simulink library "LiftMotionControlLibrary"  (R2021b)
settings: Solver=VariableStepAuto  StartTime=0.0  StopTime=10.0  RelTol=1e-3
values from neighbouring files (symbols this model uses):
  floor_height = 3    [test_motion_law.m]
  gearbox = 1    [test_motion_law.m]
  max_load = 800    [test_motion_law.m]
  MaxAcc = 1    [test_motion_law.m]
  MaxJerk = 1    [test_motion_law.m]
  MaxVel = 2    [test_motion_law.m]
  MinVel = 0.2    [test_motion_law.m]
  motion_profile = 1    [test_motion_law.m]
  num_floors = 20    [test_motion_law.m]
  proximity_distance = 1    [test_motion_law.m]
  Ts = 1e-3    (= 0.001)    [test_motion_law.m]
undefined symbols (not defined in the file or in its folder): cabin_offset, Rp, sensor_height, waiting_time_close_brake, waiting_time_close_door, waiting_time_open_brake, waiting_time_open_door, waiting_time_steady_state
libraries: $bdroot x2, cstblocks x1
settings Model: Creator=manue  LastModifiedBy=manue

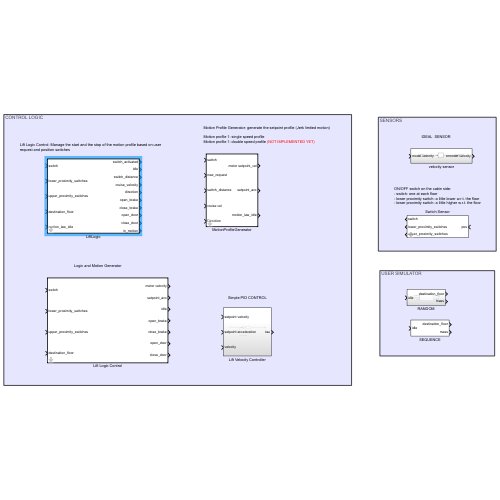
[thumbnail: Simulink's stored preview of the top-level diagram]
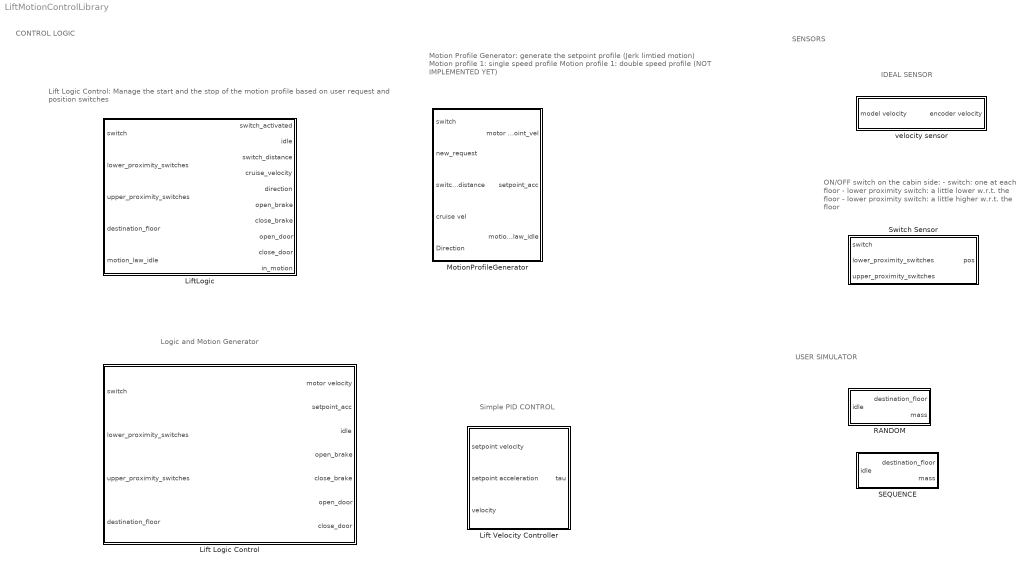
== system LiftMotionControlLibrary ==
  note: Logic and Motion Generator
  note: IDEAL SENSOR
  note: ON/OFF switch on the cabin side:
      | - switch: one at each floor
      | - lower proximity switch: a little lower w.r.t. the floor
      | - lower proximity switch: a little higher w.r.t. the floor
  note: SENSORS
  note: CONTROL LOGIC
  note: Simple PID CONTROL
  note: Motion Profile Generator: generate the setpoint profile (Jerk limtied motion)
      |
      | Motion profile 1: single speed profile
      | Motion profile 1: double speed profile (NOT IMPLEMENTED YET)
  note: Lift Logic Control: Manage the start and the stop of the motion profile based on user request and position switches
  note: USER SIMULATOR
  Lift Logic Control : Subsystem  TreatAsAtomicUnit=on  SystemSampleTime=Ts  mask{floor_height=floor_height, num_floors=num_floors, sensor_height=sensor_height, proximity_distance=proximity_distance, MinVel=MinVel, MaxVel=MaxVel, Ts=Ts, MaxAcc=MaxAcc, MaxJerk=MaxJerk, gearbox=gearbox, cabin_offset=cabin_offset, Rp=Rp, motion_profile=Profile 1: single speed, waiting_time_open_door=waiting_time_open_door, waiting_time_close_door=waiting_time_close_door, waiting_time_open_brake=waiting_time_open_brake, waiting_time_close_brake_copy=waiting_time_close_brake, waiting_time_steady_state=waiting_time_steady_state}
      mask prompts: floor_height "Floor Height"; num_floors "Number of floors"; sensor_height "Sensor Height"; proximity_distance "Distance of the proximity switches"; MinVel "Lower lift velocity"; MaxVel "Maximum lift velocity"; Ts "Sample period"; MaxAcc "Maximum acceleration"; MaxJerk "Maximum Jerk"; gearbox "gearbox ratio"; cabin_offset "Cabin offset compensation"; Rp "Pulley Radius"; motion_profile "Type of Motion Profile"; waiting_time_open_door "Time to open doors"; waiting_time_close_door "Time to close doors"; waiting_time_open_brake "Time to open brake"; waiting_time_close_brake_copy "Time to close brake"; waiting_time_steady_state "Time to reach zero velocity"
      mask TypeOptions motion_profile: Profile 1: single speed | Profile 2: multiple speed (not implmeneted yet)
  Lift Velocity Controller : Subsystem
  LiftLogic : Subsystem  TreatAsAtomicUnit=on  SystemSampleTime=Ts  mask{floor_height=floor_height, num_floors=num_floors, sensor_height=sensor_height, proximity_distance=proximity_distance, motion_profile=motion_profile, MinVel=MinVel, MaxVel=MaxVel, cabin_offset=cabin_offset, Ts=Ts, waiting_time_open_door=waiting_time_open_door, waiting_time_close_door=waiting_time_close_door, waiting_time_open_brake=waiting_time_open_brake, waiting_time_close_brake=waiting_time_close_brake, waiting_time_steady_state=waiting_time_steady_state}
      mask prompts: floor_height "Floor Height"; num_floors "Number of floors"; sensor_height "Sensor Height"; proximity_distance "Distance of the proximity switches"; motion_profile "Type of Motion Profile"; MinVel "Lower lift velocity"; MaxVel "Maximum lift velocity"; cabin_offset "Cabin offset compensation"; Ts "Sample period"; waiting_time_open_door "Time to open the doors"; waiting_time_close_door "Time to close the doors"; waiting_time_open_brake "Time to open the brake"; waiting_time_close_brake "Time to close the brake"; waiting_time_steady_state "Time to reach zero velocity"
  MotionProfileGenerator : Subsystem  TreatAsAtomicUnit=on  SystemSampleTime=Ts  mask{MaxAcc=MaxAcc, MaxJerk=MaxJerk, Ts=Ts, gearbox=gearbox, Rp=Rp, motion_profile=motion_profile}
      mask prompts: MaxAcc "Maximum acceleration"; MaxJerk "MaximumJerk"; Ts "Sample period"; gearbox "gearbox ratio"; Rp "Pulley Radius"; motion_profile "Type of Motion profile"
  RANDOM : Subsystem
  SEQUENCE : Subsystem  mask{sequence=[5 10 15 10]}
      mask prompts: sequence "Floor sequence"
  Switch Sensor : Subsystem  mask{floor_height=floor_height, num_floors=num_floors, proximity_distance=proximity_distance, sensor_height=sensor_height}
      mask prompts: floor_height "Floor Height"; num_floors "Number of floors"; proximity_distance "Distance of the proximity switches"; sensor_height "Sensor Height"
      mask help: switches return -1 if not activated, the number of floor if activated
  velocity sensor : Subsystem

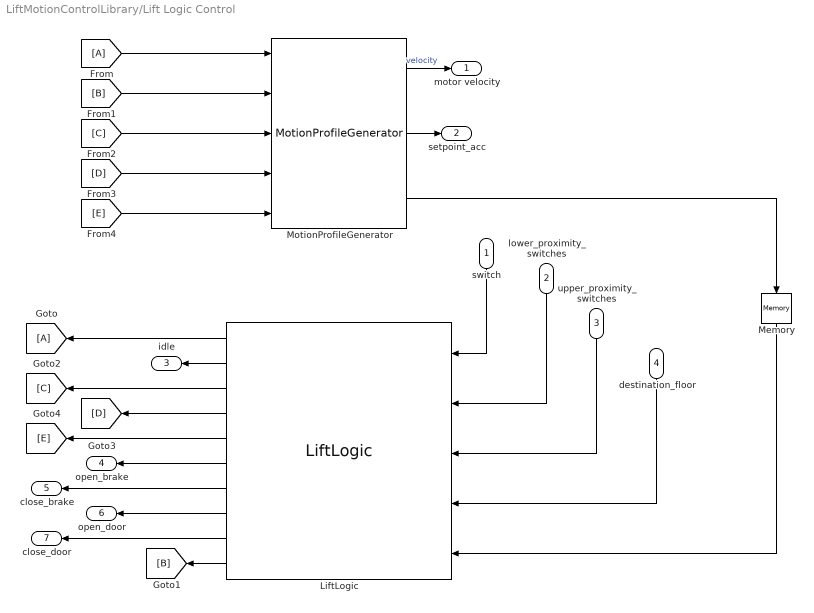
== system LiftMotionControlLibrary/Lift Logic Control ==
  switch : Inport
  lower_proximity_switches : Inport  Port=2
  upper_proximity_switches : Inport  Port=3
  destination_floor : Inport  Port=4
  LiftLogic : $bdroot/LiftLogic  floor_height=floor_height  num_floors=num_floors  sensor_height=sensor_height  proximity_distance=proximity_distance  motion_profile=motion_profile  MinVel=MinVel  MaxVel=MaxVel  cabin_offset=cabin_offset  Ts=Ts  waiting_time_open_door=waiting_time_open_door  waiting_time_close_door=waiting_time_close_door  waiting_time_open_brake=waiting_time_open_brake  waiting_time_close_brake=waiting_time_close_brake  waiting_time_steady_state=waiting_time_steady_state
  Memory : Memory  InheritSampleTime=on
  MotionProfileGenerator : $bdroot/MotionProfileGenerator  MaxAcc=MaxAcc  MaxJerk=MaxJerk  Ts=Ts  gearbox=gearbox  Rp=Rp  motion_profile=motion_profile
  motor velocity : Outport
  setpoint_acc : Outport  Port=2
  idle : Outport  Port=3
  open_brake : Outport  Port=4
  close_brake : Outport  Port=5
  open_door : Outport  Port=6
  close_door : Outport  Port=7
  wires:
  [E] -> MotionProfileGenerator/5
  LiftLogic/5 -> [E]
  [D] -> MotionProfileGenerator/4
  LiftLogic/4 -> [D]
  [C] -> MotionProfileGenerator/3
  LiftLogic/3 -> [C]
  LiftLogic/2 -> idle/1
  [A] -> MotionProfileGenerator/1
  LiftLogic/1 -> [A]
  Memory/1 -> LiftLogic/5
  MotionProfileGenerator/3 -> Memory/1
  destination_floor/1 -> LiftLogic/4
  lower_proximity_switches/1 -> LiftLogic/2
  switch/1 -> LiftLogic/1
  MotionProfileGenerator/1 -> motor velocity/1  "velocity"
  MotionProfileGenerator/2 -> setpoint_acc/1
  upper_proximity_switches/1 -> LiftLogic/3
  [B] -> MotionProfileGenerator/2
  LiftLogic/10 -> [B]
  LiftLogic/9 -> close_door/1
  LiftLogic/8 -> open_door/1
  LiftLogic/7 -> close_brake/1
  LiftLogic/6 -> open_brake/1

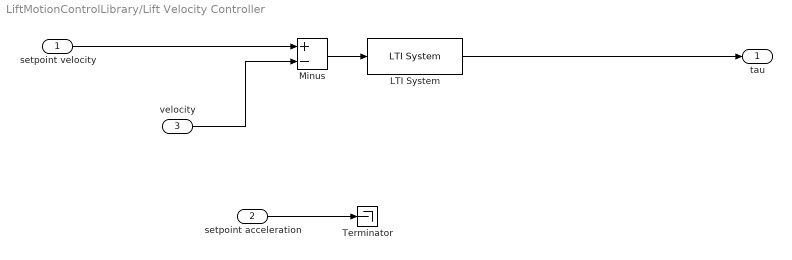
== system LiftMotionControlLibrary/Lift Velocity Controller ==
  setpoint velocity : Inport
  setpoint acceleration : Inport  Port=2
  velocity : Inport  Port=3
  LTI System : cstblocks/LTI System  sys=ctrl  IC=[]
  Minus : Sum  Inputs=+-
  Terminator : Terminator
  tau : Outport
  wires:
  setpoint acceleration/1 -> Terminator/1
  velocity/1 -> Minus/2
  Minus/1 -> LTI System/1
  setpoint velocity/1 -> Minus/1
  LTI System/1 -> tau/1

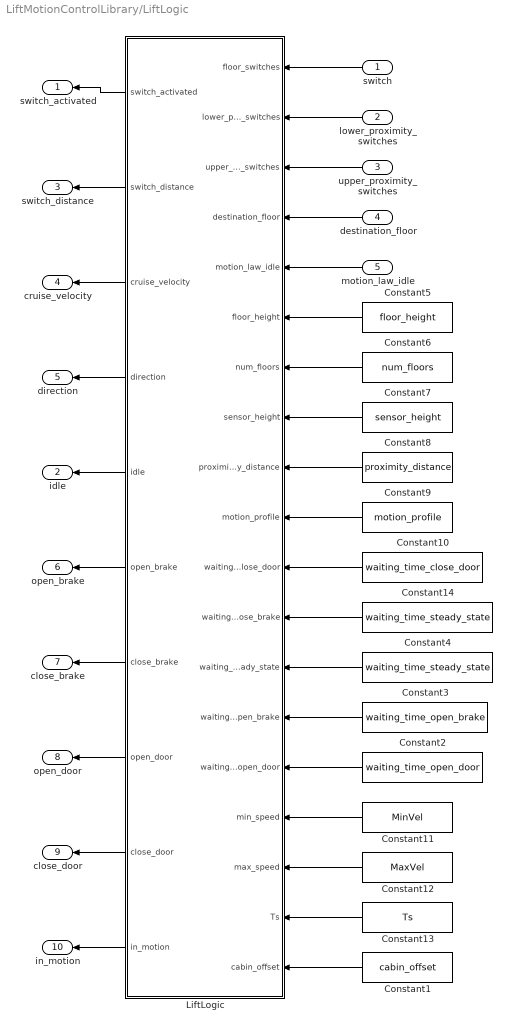
== system LiftMotionControlLibrary/LiftLogic ==
  switch : Inport
  lower_proximity_switches : Inport  Port=2
  upper_proximity_switches : Inport  Port=3
  destination_floor : Inport  Port=4
  motion_law_idle : Inport  Port=5
  Constant1 : Constant  Value=cabin_offset
  Constant10 : Constant  Value=waiting_time_close_door
  Constant11 : Constant  Value=MinVel
  Constant12 : Constant  Value=MaxVel
  Constant13 : Constant  Value=Ts
  Constant14 : Constant  Value=waiting_time_steady_state  VectorParams1D=off
  Constant2 : Constant  Value=waiting_time_open_door
  Constant3 : Constant  Value=waiting_time_open_brake
  Constant4 : Constant  Value=waiting_time_steady_state  VectorParams1D=off
  Constant5 : Constant  Value=floor_height
  Constant6 : Constant  Value=num_floors
  Constant7 : Constant  Value=sensor_height
  Constant8 : Constant  Value=proximity_distance
  Constant9 : Constant  Value=motion_profile
  LiftLogic : MATLAB Function  TreatAsAtomicUnit=on
  switch_activated : Outport  OutDataTypeStr=boolean
  idle : Outport  Port=2
  switch_distance : Outport  Port=3
  cruise_velocity : Outport  Port=4
  direction : Outport  Port=5
  open_brake : Outport  Port=6
  close_brake : Outport  Port=7
  open_door : Outport  Port=8
  close_door : Outport  Port=9
  in_motion : Outport  Port=10
  wires:
  LiftLogic/1(switch_activated) -> switch_activated/1
  Constant5/1 -> LiftLogic/6(floor_height)
  Constant11/1 -> LiftLogic/16(min_speed)
  Constant1/1 -> LiftLogic/19(cabin_offset)
  switch/1 -> LiftLogic/1(floor_switches)
  Constant12/1 -> LiftLogic/17(max_speed)
  Constant7/1 -> LiftLogic/8(sensor_height)
  Constant10/1 -> LiftLogic/11(waiting_time_close_door)
  LiftLogic/3(cruise_velocity) -> cruise_velocity/1
  upper_proximity_switches/1 -> LiftLogic/3(upper_proximity_switches)
  Constant13/1 -> LiftLogic/18(Ts)
  Constant8/1 -> LiftLogic/9(proximity_distance)
  motion_law_idle/1 -> LiftLogic/5(motion_law_idle)
  LiftLogic/4(direction) -> direction/1
  LiftLogic/5(idle) -> idle/1
  Constant6/1 -> LiftLogic/7(num_floors)
  LiftLogic/2(switch_distance) -> switch_distance/1
  destination_floor/1 -> LiftLogic/4(destination_floor)
  lower_proximity_switches/1 -> LiftLogic/2(lower_proximity_switches)
  Constant9/1 -> LiftLogic/10(motion_profile)
  Constant2/1 -> LiftLogic/15(waiting_time_open_door)
  Constant14/1 -> LiftLogic/12(waiting_time_close_brake)
  Constant4/1 -> LiftLogic/13(waiting_time_steady_state)
  Constant3/1 -> LiftLogic/14(waiting_time_open_brake)
  LiftLogic/6(open_brake) -> open_brake/1
  LiftLogic/7(close_brake) -> close_brake/1
  LiftLogic/8(open_door) -> open_door/1
  LiftLogic/9(close_door) -> close_door/1
  LiftLogic/10(in_motion) -> in_motion/1

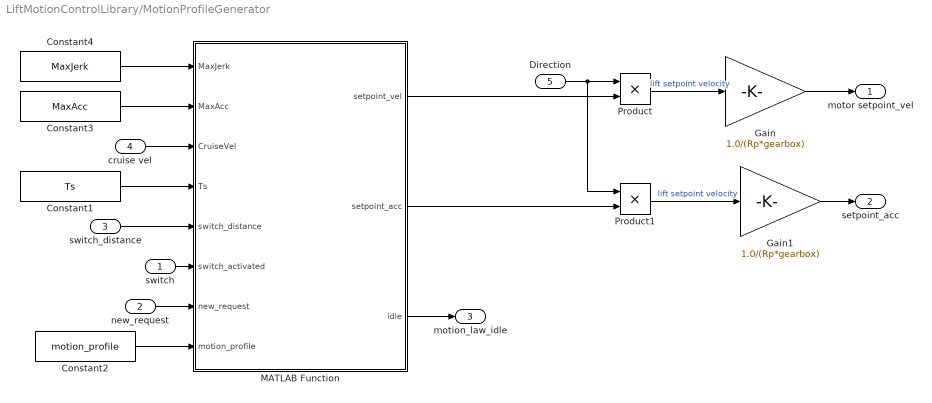
== system LiftMotionControlLibrary/MotionProfileGenerator ==
  switch : Inport
  new_request : Inport  Port=2
  switch_distance : Inport  Port=3
  cruise vel : Inport  Port=4
  Direction : Inport  Port=5
  Constant1 : Constant  Value=Ts
  Constant2 : Constant  Value=motion_profile
  Constant3 : Constant  Value=MaxAcc
  Constant4 : Constant  Value=MaxJerk
  Gain : Gain  Gain=1.0/(Rp*gearbox)
  Gain1 : Gain  Gain=1.0/(Rp*gearbox)
  MATLAB Function : MATLAB Function  TreatAsAtomicUnit=on
  Product : Product
  Product1 : Product
  motor setpoint_vel : Outport
  setpoint_acc : Outport  Port=2
  motion_law_idle : Outport  Port=3
  wires:
  new_request/1 -> MATLAB Function/7(new_request)
  MATLAB Function/3(idle) -> motion_law_idle/1
  Gain/1 -> motor setpoint_vel/1
  Product/1 -> Gain/1  "lift setpoint velocity"
  Direction/1 -> Product1/1, Product/1
  MATLAB Function/1(setpoint_vel) -> Product/2
  MATLAB Function/2(setpoint_acc) -> Product1/2
  Constant4/1 -> MATLAB Function/1(MaxJerk)
  Constant3/1 -> MATLAB Function/2(MaxAcc)
  switch/1 -> MATLAB Function/6(switch_activated)
  Constant1/1 -> MATLAB Function/4(Ts)
  switch_distance/1 -> MATLAB Function/5(switch_distance)
  cruise vel/1 -> MATLAB Function/3(CruiseVel)
  Gain1/1 -> setpoint_acc/1
  Product1/1 -> Gain1/1  "lift setpoint velocity"
  Constant2/1 -> MATLAB Function/8(motion_profile)

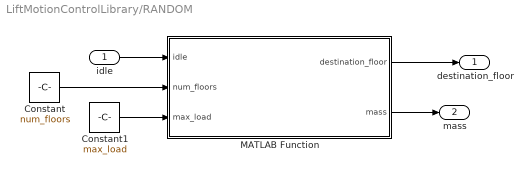
== system LiftMotionControlLibrary/RANDOM ==
  idle : Inport
  Constant : Constant  Value=num_floors
  Constant1 : Constant  Value=max_load
  MATLAB Function : MATLAB Function  TreatAsAtomicUnit=on
  destination_floor : Outport  OutDataTypeStr=double
  mass : Outport  Port=2  OutDataTypeStr=double
  wires:
  idle/1 -> MATLAB Function/1(idle)
  Constant/1 -> MATLAB Function/2(num_floors)
  Constant1/1 -> MATLAB Function/3(max_load)
  MATLAB Function/1(destination_floor) -> destination_floor/1
  MATLAB Function/2(mass) -> mass/1

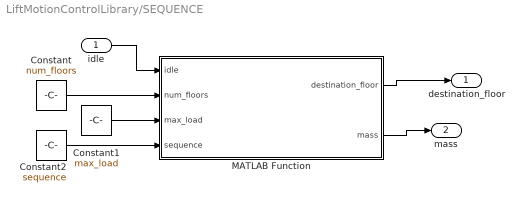
== system LiftMotionControlLibrary/SEQUENCE ==
  idle : Inport
  Constant : Constant  Value=num_floors
  Constant1 : Constant  Value=max_load
  Constant2 : Constant  Value=sequence
  MATLAB Function : MATLAB Function  TreatAsAtomicUnit=on
  destination_floor : Outport  OutDataTypeStr=double
  mass : Outport  Port=2  OutDataTypeStr=double
  wires:
  MATLAB Function/2(mass) -> mass/1
  MATLAB Function/1(destination_floor) -> destination_floor/1
  Constant1/1 -> MATLAB Function/3(max_load)
  Constant/1 -> MATLAB Function/2(num_floors)
  idle/1 -> MATLAB Function/1(idle)
  Constant2/1 -> MATLAB Function/4(sequence)

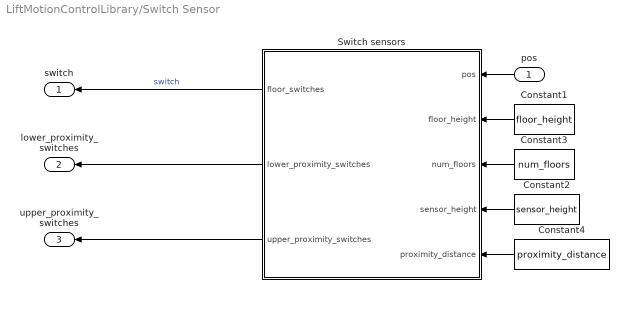
== system LiftMotionControlLibrary/Switch Sensor ==
  pos : Inport
  Constant1 : Constant  Value=floor_height
  Constant2 : Constant  Value=sensor_height
  Constant3 : Constant  Value=num_floors
  Constant4 : Constant  Value=proximity_distance
  Switch sensors : MATLAB Function  TreatAsAtomicUnit=on
  switch : Outport
  lower_proximity_switches : Outport  Port=2
  upper_proximity_switches : Outport  Port=3
  wires:
  Switch sensors/1(floor_switches) -> switch/1  "switch"
  pos/1 -> Switch sensors/1(pos)
  Constant1/1 -> Switch sensors/2(floor_height)
  Constant3/1 -> Switch sensors/3(num_floors)
  Constant4/1 -> Switch sensors/5(proximity_distance)
  Constant2/1 -> Switch sensors/4(sensor_height)
  Switch sensors/3(upper_proximity_switches) -> upper_proximity_switches/1
  Switch sensors/2(lower_proximity_switches) -> lower_proximity_switches/1

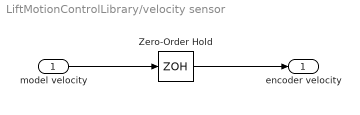
== system LiftMotionControlLibrary/velocity sensor ==
  model velocity : Inport
  Zero-Order Hold : ZeroOrderHold  SampleTime=Ts
  encoder velocity : Outport
  wires:
  model velocity/1 -> Zero-Order Hold/1
  Zero-Order Hold/1 -> encoder velocity/1

== matlab function LiftMotionControlLibrary/SEQUENCE/MATLAB Function ==
  data: idle input; destination_floor output; num_floors input; max_load input; mass output double; sequence input
function [destination_floor,mass]  = simulatePeople(idle,num_floors,max_load,sequence)

persistent destination_internal mass_internal idx_sequence
if isempty(destination_internal)
    destination_internal=0;
    mass_internal=0.0;
    idx_sequence=1;
end

if (idle)
    if (idx_sequence>length(sequence))
        idx_sequence=1;
    end
    destination_internal=sequence(idx_sequence);
    % mass variation for each cycles +/- 400 kg
    mass_internal=min(max(0,mass_internal+(2*rand-1)*80*5),max_load); 
    idx_sequence=idx_sequence+1;

end
destination_floor=destination_internal;
mass=mass_internal;

== matlab function LiftMotionControlLibrary/Switch Sensor/Switch sensors ==
  data: pos input; floor_switches output; floor_height input; num_floors input; sensor_height input; proximity_distance input; lower_proximity_switches output; upper_proximity_switches output
function [floor_switches,lower_proximity_switches,upper_proximity_switches]=SwitchPosition(pos,floor_height,num_floors,sensor_height,proximity_distance)
% switches return -1 if not activated, the number of floor if activated

floor_switches=-1;
lower_proximity_switches=-1;
upper_proximity_switches=-1;
for floor_index=0:num_floors

    % floor switch
    switch_pos=floor_index*floor_height;
    if (pos<=switch_pos && (pos+sensor_height)>=(switch_pos))
        floor_switches=floor_index;
    end

    % lower proximity switch
    switch_pos=floor_index*floor_height+sensor_height-proximity_distance;
    if (pos<=switch_pos && (pos+sensor_height)>=(switch_pos))
        lower_proximity_switches=floor_index;
    end
    
    % upper proximity switch
    switch_pos=floor_index*floor_height+proximity_distance;
    if (pos<=switch_pos && (pos+sensor_height)>=(switch_pos))
        upper_proximity_switches=floor_index;
    end
end

== matlab function LiftMotionControlLibrary/MotionProfileGenerator/MATLAB Function ==
  data: MaxJerk input; setpoint_vel output; MaxAcc input; CruiseVel input; Ts input; switch_distance input; switch_activated input; setpoint_acc output; new_request input; idle output boolean; motion_profile input
function [setpoint_vel,setpoint_acc,idle]=MotionLaw(MaxJerk,MaxAcc,CruiseVel,Ts,switch_distance,switch_activated,new_request,motion_profile)

persistent state vel acc pos
if isempty(state)
    state=0;
    vel=0;
    acc=0;
    pos=0;
end

% compute deceleration distance: 
% case 1: the maximum acceleration is reached
% case 2: the maximum acceleration is not reached
if (CruiseVel^(1/2)*MaxJerk^(1/2)>MaxAcc) % case 1
    deceleration_distance=(CruiseVel*(MaxAcc^2 + CruiseVel*MaxJerk))/(2*MaxAcc*MaxJerk);
else % case 2
    deceleration_distance =CruiseVel^(3/2)/MaxJerk^(1/2);
end

if (state==1)  %increase acceleration
    jerk=MaxJerk;
elseif (state==2) % max acceleration
    jerk=0;
elseif (state==3) % decrease acceleration
    jerk=-MaxJerk;
elseif (state==4) % keep cruise velocity
    jerk=0;
elseif (state==5) % kep cruise velocity, switch has been triggered
    jerk=0;
elseif (state==6) % decrease acceleration (to slow down speed)
    jerk=-MaxJerk;
elseif (state==7) % max negative acceleration (to slow down speed)
    jerk=0;
elseif (state==8) % increase acceleration (to return to null acceleration)
    jerk=MaxJerk;

elseif state==11 % decrease acceleration (to reach low speed)  PROFILE==2
    jerk=-MaxJerk;
elseif state==12 % max negative acceleration (to reach low speed)  PROFILE==2
    jerk=0;
elseif state==13 % increase acceleration (to return to null acceleration)  PROFILE==2
    jerk=MaxJerk;
elseif (state==14) % keep cruise velocity
    jerk=0;
else % steaty-state case
    jerk=0;
    vel=0;
    acc=0;

end


pos=pos+vel*Ts+0.5*acc*Ts^2+1.0/6.0*jerk*Ts^3; % traveled distance
vel=vel+acc*Ts+0.5*Ts*Ts*jerk; % velocity
acc=acc+Ts*jerk; % acceleration

limit_velocity=CruiseVel-acc^2/(2*MaxJerk); % velocity limit to start removing accelaration to reach cruise velocity
limit_velocity_profile2=CruiseVel+acc^2/(2*MaxJerk); % velocity limit to start removing accelaration to reach low velocity
limit_velocity_final=acc^2/(2*MaxJerk); % velocity limit to start removing accelaration to reach null velocity

%% state machine transition 
if (state==0 && new_request)
    state=1;
elseif (state==1 && acc>=MaxAcc) % max acceleration reached
    state=2;
    acc=min(acc,MaxAcc);
elseif ((state==2 || state==1) && vel>=limit_velocity) % limit velocity reached  (cruise velocity will be reached soon)
    state=3;
elseif (state==3 && acc<=0) % null acceleration reached
    state=4;
    acc=0;
elseif (state==4 && switch_activated) % switch has been triggered
    if (motion_profile==1)
        state=5;
    else
        state=11;
    end
    pos=0;
elseif (state==5 && pos>=(switch_distance-deceleration_distance)) % time to slow down
    state=6;
elseif (state==6 && acc<=-MaxAcc) % negative max acceleration reached
    state=7;
    acc=max(acc,-MaxAcc);
elseif ((state==7 || state==6) && vel<=limit_velocity_final) % limit acceleration to stop motion is reached
    state=8;
elseif (state==8 && vel<=0) % steady state reached
    state=0;
    vel=0;
    acc=0;


elseif (state==11 && acc<=-MaxAcc)
    state=12;
    acc=max(acc,-MaxAcc);
elseif ((state==11 || state==12)  && vel<=limit_velocity_profile2)
    state=13;
elseif (state==13 && vel<=CruiseVel) % steady state reached
    state=14;
    vel=CruiseVel;
    acc=0;
elseif (state==14 && switch_activated) % switch has been triggered
    state=5;
    pos=0;
end

idle=state==0;
setpoint_vel=vel;
setpoint_acc=acc;

== matlab function LiftMotionControlLibrary/LiftLogic/LiftLogic ==
  data: floor_switches input; switch_activated output; lower_proximity_switches input; upper_proximity_switches input; destination_floor input; motion_law_idle input; floor_height input; num_floors input; sensor_height input; proximity_distance input; motion_profile input; waiting_time_close_door input; waiting_time_close_brake input; waiting_time_steady_state input; waiting_time_open_brake input; waiting_time_open_door input; min_speed input; max_speed input; Ts input; switch_distance output; cruise_velocity output; direction output; idle output; cabin_offset input; open_brake output; close_brake output; open_door output; close_door output; in_motion output
function [switch_activated,switch_distance,cruise_velocity,direction,idle,open_brake,close_brake,open_door,close_door,in_motion]=LiftLogic(floor_switches,...
    lower_proximity_switches,...
    upper_proximity_switches,...
    destination_floor,...
    motion_law_idle,...
    floor_height,...
    num_floors,...
    sensor_height,...
    proximity_distance,...
    motion_profile,...
    waiting_time_close_door,...
    waiting_time_close_brake,...
    waiting_time_steady_state,...
    waiting_time_open_brake,...
    waiting_time_open_door,...
    min_speed,...
    max_speed,...
    Ts,...
    cabin_offset)

persistent req_floor state start_floor time cruise_velocity_internal direction_internal open_brake_cmd_internal open_door_internal close_brake_cmd_internal close_door_internal

if isempty(req_floor)
    if floor_switches>=0 % lift is parked in one floor at the beginning
        start_floor=floor_switches;
    else % abnormal behaviour lift in not parked in one floor at the beginning, go to the last floor
        start_floor=-1;
        destination_floor=num_floors;
    end
    req_floor=start_floor;
    state=0;
    time=0;
    cruise_velocity_internal=0;
    direction_internal=0;

    open_brake_cmd_internal=true;
    open_door_internal=false;
    close_brake_cmd_internal=false;
    close_door_internal=false;
end

switch_activated=false;
switch_distance=0;
idle=false;
% state:
% 0 IDLE
% 1 close the door
% 2 open the break
% 3 LIFT IS MOVING
% 4 LIFT IS MOVING AT LOW VELOCITY
% 5 STOPPING
% 6 close the break
% 7 open the door

% ACTIONS

if state==3
    if (direction_internal>0)
        switch_activated=floor_switches==(req_floor-1); % the top of the cabin reaches the floor switch
        switch_distance=floor_height+sensor_height+cabin_offset;
    else
        switch_activated=floor_switches==(req_floor+1); % the bottom of the cabin reaches the upper floor switch
        switch_distance=floor_height+cabin_offset;
    end
elseif state==4
    if (direction_internal>0)
        switch_activated=lower_proximity_switches==(req_floor); % the top of the cabin reaches the floor switch
        switch_distance= proximity_distance + cabin_offset;
    else
        switch_activated=upper_proximity_switches==(req_floor); % the bottom of the cabin reaches the upper floor switch
        switch_distance=proximity_distance+cabin_offset;
    end
elseif state~=0
    time=time+Ts;
end


in_motion=false;

% TRANSITIONS
if (state==0 && (destination_floor~=start_floor))
    if ( (destination_floor>num_floors) || (destination_floor<0) )
        % you should not go here!
    else
        time=0;
        state=1;
        req_floor=destination_floor;
        close_door_internal=true;
            if abs(req_floor-start_floor)==1
                cruise_velocity_internal=min_speed;
            else
                cruise_velocity_internal=max_speed;
            end
            if (req_floor>start_floor)
                direction_internal=1;
            else
                direction_internal=-1;
            end

    end
elseif (state==1 && time>waiting_time_open_door)
    close_door_internal=false;
    time=0;
    open_brake_cmd_internal=true;
    state=2;
elseif (state==2 && time>waiting_time_open_brake)
    open_brake_cmd_internal=false;
    time=0;
    state=3;
    in_motion=true;
elseif (state==3 && motion_profile==2 && switch_activated)
    cruise_velocity_internal=min_speed;
    state=4;
elseif ( (state==3 && motion_law_idle && motion_profile==1) || (state==4 && motion_law_idle && motion_profile==2))
    state=5;
    time=0;
    start_floor=req_floor;
elseif (state==5 && time>waiting_time_steady_state)
    state=6;
    time=0;
    close_brake_cmd_internal=true;
elseif (state==6 && time>waiting_time_close_brake)
    time=0;
    open_door_internal=true;
    close_brake_cmd_internal=false;
    state=7;
elseif (state==7 && time>waiting_time_close_door)
    time=0;
    open_door_internal=true;
    state=0;
end



cruise_velocity=cruise_velocity_internal;
direction=direction_internal;
idle=state==0;
close_door=close_door_internal;
open_door=open_door_internal;
close_brake=close_brake_cmd_internal;
open_brake=open_brake_cmd_internal;

== matlab function LiftMotionControlLibrary/RANDOM/MATLAB Function ==
  data: idle input; destination_floor output; num_floors input; max_load input; mass output double
function [destination_floor,mass]  = simulatePeople(idle,num_floors,max_load)

persistent destination_internal mass_internal
if isempty(destination_internal)
    destination_internal=0;
    mass_internal=0.0;
end

if (idle)
    destination_internal=randi(num_floors+1)-1;
    % mass variation for each cycles +/- 400 kg
    mass_internal=min(max(0,mass_internal+(2*rand-1)*80*5),max_load); 

end
destination_floor=destination_internal;
mass=mass_internal;
